simulink model "pwm2_PWM_task"  (Simulink 3.00)
libraries: mathlib x1, reglib x1, arclib x1

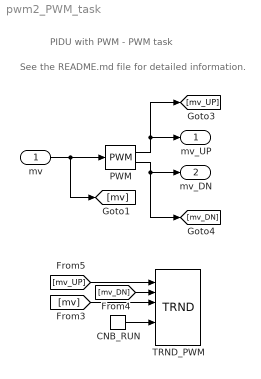
== system pwm2_PWM_task ==
  note: See the README.md file for detailed information.
  note: PIDU with PWM - PWM task
  mv : Inport  Port=1
  CNB_RUN : mathlib/CNB  YCN=on
  PWM : reglib/PWM  pertm=2  dtime=0.1  btime=0.1  offtime=0.1  asyfac=1  SYNCH=off
  TRND_PWM : arclib/TRND  n=3  l=100  btype=8  ptype1=1: Store  ptype2=1: Store  ptype3=1: Store  ptype4=1: Store  pfac=1  afac=0  arc=0  id=2  Title=Trend Title  timesrc=1
  mv_UP : Outport  Port=1
  mv_DN : Outport  Port=2
  wires:
  CNB_RUN/1 -> TRND_PWM/5
  [mv] -> TRND_PWM/3
  [mv_DN] -> TRND_PWM/2
  [mv_UP] -> TRND_PWM/1
  PWM/1 -> [mv_UP], mv_UP/1
  PWM/2 -> [mv_DN], mv_DN/1
  mv/1 -> [mv], PWM/1
